simulink library "lib_controls"  (Simulink 7.9)
settings: Solver=ode45  SolverMode=SingleTasking  StartTime=0.0  StopTime=10.0  RelTol=1e-3
undefined symbols (not defined in the file or in its folder): amb_tmp, cs_charge_deplete_bool, cs_charge_pwr, cs_charge_trq, cs_clt_tmp, cs_decel_fc_off, cs_decel_regen_threshold, cs_dl_assist_trq_threshold, cs_dl_regen_trq_threshold, cs_electric_decel_spd, cs_electric_launch_spd, cs_electric_launch_spd_hi, cs_electric_launch_spd_lo, cs_eng_min_spd, cs_eng_on_soc, cs_fc_init_state, cs_fc_max_pwr_frac, cs_fc_min_pwr_frac, cs_fc_on, cs_fc_pwr_opt, cs_fc_spd_opt, cs_fuzzy_fuel_mode, cs_hi_soc, cs_hi_trq_frac, cs_lo_soc, cs_lo_trq_frac, cs_max_gc_spd, cs_max_pwr, cs_max_pwr_fall_rate, cs_max_pwr_rise_rate, cs_mc_assist_max_frac, cs_mc_assist_min_frac, cs_mc_assist_slope, cs_mc_regen_max_frac, cs_mc_regen_min_frac, cs_mc_regen_slope, cs_mean_eff, cs_mean_eff_bool, cs_min_gc_spd, cs_min_off_time, cs_min_pwr, cs_min_trq_frac, cs_mph_avg_time, cs_off_trq_frac, cs_plot_output, cs_pwr, cs_regen_avg_time, cs_scale_factor, cs_shutoff, cs_soc_range, cs_spd, cs_target_soc, cs_trq_to_soc_factor, cvt_locus_pwr, cvt_locus_spd, cyc_mph, enable_sim_stop_distance, enable_sim_stop_max_spd, enable_sim_stop_speed, enable_sim_stop_time ... (+110)
libraries: lib_controls x124, simulink3 x13, simulink x5, lib_etc x1
(part 1 of 17)
settings Model: Creator=mokeefe  LastModifiedBy=mokeefe
settings Model: ModifiedComment=|
  | mokeefe -- Fri Mar 23 16:02:54 2012 -- Version 1.480
  | Updated all instances of @1 variables in key-on block masks to use the variable name ("t" in all cases).
settings Model: ModifiedHistory=|
  | mokeefe -- Fri Mar 23 16:02:54 2012 -- Version 1.480
  | Updated all instances of @1 variables in key-on block masks to use the variable name ("t" in all cases).
  | 
  | mokeefe -- Fri Mar 23 15:55:42 2012 -- Version 1.479
  | Fixed mask issues -- key_on @1 to "t"
  | 
  | mokeefe -- Fri Mar 23 15:20:48 2012 -- Version 1.478
  | updated maks variable from @1 to variable name.
  | 
  | mokeefe -- Fri Mar 23 14:57:12 2012 -- Version 1.477
  | 
  | 
  | mokeefe -- Fri Mar 23 14:56:40 2012 -- Version 1.476
  | Updated <vc> conv cvt/engine control/key_on mask initialization from @1 to variable name.
  | 
  | mokeefe -- Fri Mar 23 14:35:59 2012 -- Version 1.475
  | Updated mask variable from @1 to variable name.
  | 
  | mokeefe -- Fri Mar 23 09:48:31 2012 -- Version 1.474
  | Fixed MaskInitiation string of block 'engine control/key_on' which used mask variables by reference (@1) vs by variable name.
  | 
  | ssprik -- Fri Oct 10 08:40:34 2003 -- Version 1.473
  | added goto tag for F_rear_brake_req
  | 
  | ssprik -- Thu Oct 09 15:11:40 2003 -- Version 1.472
  | added F_rear_brake_req   goto
  | 
  | tmarkel -- Fri Mar 07 09:53:07 2003 -- Version 1.471
  | 
  | added logic to allow user to keep the engine on during a drive cycle unless the key if off or the engine has been manually disabled
  | 
  | tmarkel -- Fri Mar 07 09:43:58 2003 -- Version 1.470
  | 
  | added an override bool to keep engine on at all times
  | 
  | 
  | tmarkel -- Mon Mar 03 14:14:43 2003 -- Version 1.469
  | 
  | updated traction control block in all vehicle control blocks to 2 axle version
  | 
  | tmarkel -- Mon Mar 03 14:07:59 2003 -- Version 1.468
  | 
  | added output from blocks for rear params from traction blocks in all vehicle control blocks
  | 
  | temp solution - added grounds as inputs to the brake controller for rear drivetrain output to eliminate warnings
  | 
  | 
  | 
  | 
  | tmarkel -- Mon Mar 03 12:40:46 2003 -- Version 1.467
  | 
  | 
  | tmarkel -- Mon Mar 03 12:37:51 2003 -- Version 1.466
  | removed extra traction control model from conv.
  | 
  | tmarkel -- Mon Mar 03 12:29:10 2003 -- Version 1.465
  | 
  | updated traction control config subsystem to be two axle model
  | 
  | tmarkel -- Mon Feb 24 16:12:37 2003 -- Version 1.464
  | updated j2452 model for 2 axles
  | 
  | abrooker -- Thu Feb 20 14:21:28 2003 -- Version 1.463
  | 
  | 
  | mokeefe -- Wed Feb 19 08:45:17 2003 -- Version 1.462
  | 
  | 
  | mokeefe -- Wed Feb 19 08:43:58 2003 -- Version 1.461
  | 
  | 
  | tmarkel -- Fri Feb 14 10:10:01 2003 -- Version 1.460
  | 
  | 
  | tmarkel -- Fri Feb 14 10:08:23 2003 -- Version 1.459
  | 
  | 
  | tmarkel -- Thu Feb 13 12:55:41 2003 -- Version 1.458
  | 
  | 
  | tmarkel -- Thu Feb 13 12:32:44 2003 -- Version 1.457
  | 
  | 
  | tmarkel -- Wed Feb 12 15:47:27 2003 -- Version 1.456
  | fixed one more broken link
  | 
  | tmarkel -- Wed Feb 12 15:29:50 2003 -- Version 1.455
  | updated conv controller to include front/rear traction model
  | 
  | 
  | tmarkel -- Wed Feb 12 15:07:56 2003 -- Version 1.454
  | fixed broken link to lib_controls_2axle
  | 
  | tmarkel -- Wed Feb 12 14:32:44 2003 -- Version 1.453
  | fixed bad link errors
  | 
  | tmarkel -- Wed Feb 12 09:39:27 2003 -- Version 1.452
  | 
  | Added the traction control blocks for a front/rear traction system to the subsystem box
  | 
  | 
  | bjeanner -- Thu Dec 26 09:42:29 2002 -- Version 1.451
  | add three new parameters: allowing calcultion of equivallent ESS function with mean efficiency; plus plotting results parameter
  | 
  | 
  | bjeanner -- Thu Dec 12 14:52:52 2002 -- Version 1.450
  | 
  | 
  | bjeanner -- Tue Dec 10 14:49:05 2002 -- Version 1.449
  | 
  | 
  | bjeanner -- Tue Dec 10 13:14:31 2002 -- Version 1.448
  | 
  | 
  | bjeanner -- Tue Dec 10 11:50:56 2002 -- Version 1.447
  | 
  | 
  | bjeanner -- Tue Dec 10 11:41:01 2002 -- Version 1.446
  | 
  | 
  | bjeanner -- Tue Dec 10 11:30:40 2002 -- Version 1.445
  | 
  | 
  | bjeanner -- Tue Dec 10 11:29:40 2002 -- Version 1.444
  | 
  | 
  | bjeanner -- Tue Dec 10 11:10:40 2002 -- Version 1.443
  | 
  | 
  | bjeanner -- Tue Dec 10 10:31:25 2002 -- Version 1.442
  | 
  | 
  | bjeanner -- Tue Dec 10 10:30:04 2002 -- Version 1.441
  | 
  | 
  | bjeanner -- Tue Dec 10 10:29:36 2002 -- Version 1.440
  | 
  | 
  | bjeanner -- Tue Dec 10 10:23:30 2002 -- Version 1.439
  | 
  | 
  | bjeanner -- Tue Dec 10 09:20:40 2002 -- Version 1.438
  | 
  | 
  | bjeanner -- Tue Dec 10 09:16:26 2002 -- Version 1.437
  | Add the template for the configurable subsystem for the BD_FUELCELL control strategy.
  | Add the fuel cell adaptive control strategy
  | 
  | 
  | mokeefe -- Tue Aug 13 07:36:17 2002 -- Version 1.436
  | Making the model look "pretty"
  | 
  | mokeefe -- Tue Aug 13 07:35:11 2002 -- Version 1.435
  | changed <vc> conv cvt/cvt control to use "acc_mech_pwr_est" instead of "acc_mech_trq_est" as had been used previously (the required datum is the power and not the torque!)
  | 
  | ssprik -- Tue Apr 30 11:21:35 2002 -- Version 1.434
  | added user contributed par bal engine on  block
  | 
  | mokeefe -- Tue Apr 23 09:06:10 2002 -- Version 1.433
  | changed Insight electric assist control strategy <cs> DIRECT SPLIT/Hard Acceleration to prevent a divide by zero warning. Also added logic to prevent a torque request above the maximum achievable motor torque.
  | 
  | mokeefe -- Tue Apr 23 09:03:51 2002 -- Version 1.432
  | changed Insight electric assist control strategy <cs> DIRECT SPLIT/Hard Acceleration to prevent a divide by zero warning. Also added logic to prevent a torque request above the maximum achievable motor torque.
  | 
  | mokeefe -- Tue Apr 23 08:50:58 2002 -- Version 1.431
  | 
  | 
  | ssprik -- Thu Apr 18 14:34:50 2002 -- Version 1.430
  | 
  | 
  | ssprik -- Thu Apr 18 14:32:52 2002 -- Version 1.429
  | 
  | 
  | ssprik -- Thu Apr 18 14:06:57 2002 -- Version 1.428
  | 
  | 
  | ssprik -- Thu Apr 18 13:56:10 2002 -- Version 1.427
  | 
  | 
  | ssprik -- Thu Apr 18 13:46:32 2002 -- Version 1.426
  | 
  | 
  | kkelly -- Thu Apr 18 10:17:40 2002 -- Version 1.425
  | 
  | 
  | mokeefe -- Thu Apr 18 08:23:32 2002 -- Version 1.424
  | saving the model:
  | o "without the model browser open"
  | o with only top-level screen visible
  | o with "fit to view" enabled
  | o with "status bar" off and "toolbar" off
  | o with "prompt to update model history with each save" on
  | 
  | kkelly -- Wed Mar 27 14:57:12 2002 -- Version 1.423
  | 
  | 
  | kkelly -- Wed Mar 27 14:57:12 2002 -- Version 1.423
  | 
  | 
  | kkelly -- Wed Mar 27 14:50:41 2002 -- Version 1.422
  | 
  | 
  | kkelly -- Wed Mar 27 14:50:24 2002 -- Version 1.421
  | 
  | 
  | kkelly -- Wed Mar 27 14:26:31 2002 -- Version 1.420
  | 
  | 
  | kkelly -- Wed Mar 27 14:26:16 2002 -- Version 1.419
  | 
  | 
  | kkelly -- Wed Mar 27 14:25:54 2002 -- Version 1.418
  | 
  | 
  | kkelly -- Wed Mar 27 14:20:49 2002 -- Version 1.417
  | 
  | 
  | kkelly -- Wed Mar 27 14:18:25 2002 -- Version 1.416
  | 
  | 
  | kkelly -- Wed Mar 27 14:17:14 2002 -- Version 1.415
  | 
  | 
  | kkelly -- Wed Mar 27 14:09:18 2002 -- Version 1.414
  | 
  | 
  | kkelly -- Wed Mar 27 14:07:10 2002 -- Version 1.413
  | 
  | 
  | kkelly -- Wed Mar 27 14:04:42 2002 -- Version 1.412
  | 
  | 
  | kkelly -- Wed Mar 27 12:39:55 2002 -- Version 1.411
  | 
  | 
  | kkelly -- Wed Mar 27 12:39:35 2002 -- Version 1.410
  | 
  | 
  | kkelly -- Wed Mar 27 12:31:18 2002 -- Version 1.409
  | 
  | 
  | kkelly -- Wed Mar 27 12:12:25 2002 -- Version 1.408
  | 
  | 
  | kkelly -- Wed Mar 27 12:03:57 2002 -- Version 1.407
  | 
  | 
  | kkelly -- Wed Mar 27 12:03:11 2002 -- Version 1.406
  | Added logic to increase torque request for very hard acceleration
  | 
  | kkelly -- Wed Mar 27 11:51:32 2002 -- Version 1.405
  | Added logic to allow EM in 1st gear when torque request is high
  | 
  | kkelly -- Wed Mar 27 11:48:18 2002 -- Version 1.404
  | Added logic to allow EM at low speed with high torque request
  | 
  | kkelly -- Wed Mar 27 11:36:20 2002 -- Version 1.403
  | Added zero-torque request logic
  | 
  | kkelly -- Wed Mar 27 11:09:35 2002 -- Version 1.402
  | 
  | 
  | kkelly -- Wed Mar 27 11:07:39 2002 -- Version 1.401
  | 
  | 
  | kkelly -- Wed Mar 27 10:43:33 2002 -- Version 1.400
  | 
  | 
  | mokeefe -- Fri Mar 08 08:11:28 2002 -- Version 1.399
  | took all separate auxiliary load calculations out of the <vc> libraries. These will now use the lib_accessory goto tags (acc_mech_trq_est, acc_mech_pwr_est, acc_elec_pwr_est)
  | 
  | mokeefe -- Mon Jul 02 10:08:55 2001 -- Version 1.184
  | 
  | 
  | mokeefe -- Mon Jul 02 10:08:07 2001 -- Version 1.183
  | 
  | 
  | mokeefe -- Mon Jul 02 10:06:51 2001 -- Version 1.182
  | 
  | 
  | mokeefe -- Mon Jul 02 10:05:17 2001 -- Version 1.181
  | 
  | 
  | mokeefe -- Mon Jul 02 10:04:17 2001 -- Version 1.180
  | 
  | 
  | mokeefe -- Fri Jun 29 13:59:18 2001 -- Version 1.179
  | 
  | all <vc> blocks updated for use with variable cargo mass functionality (cargo mass by distance)--also, all <vc> top-level blocks have been "cleaned up" to look neat and organized. A sub-model library has been made and is the preferred way to do future development.
  | 
  | mokeefe -- Fri Jun 29 13:56:37 2001 -- Version 1.178
  | 
  | <vc> prius
  | 
  | mokeefe -- Fri Jun 29 13:46:29 2001 -- Version 1.177
  | 
  | 
  | mokeefe -- Fri Jun 29 13:40:43 2001 -- Version 1.176
  | 
  | 
  | mokeefe -- Fri Jun 29 13:39:38 2001 -- Version 1.175
  | 
  | <vc> series ("" "")
  | 
  | 
  | mokeefe -- Fri Jun 29 13:34:00 2001 -- Version 1.174
  | 
  | <vc> par Adaptive ("" "")
  | 
  | mokeefe -- Fri Jun 29 13:23:41 2001 -- Version 1.173
  | 
  | insight (ibid.)
  | 
  | 
  | mokeefe -- Fri Jun 29 13:15:22 2001 -- Version 1.172
  | 
  | <vc> par balanced--> veh_mass to veh_mass+veh_cargo_mass
  | 
  | 
  | mokeefe -- Fri Jun 29 13:05:39 2001 -- Version 1.171
  | 
  | 
  | mokeefe -- Fri Jun 29 12:10:12 2001 -- Version 1.170
  | 
  | finished veh_mass mods for the <vc> par cvt...
  | 
  | 
  | mokeefe -- Fri Jun 29 12:09:18 2001 -- Version 1.169
  | 
  | 
  | mokeefe -- Fri Jun 29 11:56:20 2001 -- Version 1.168
  | 
  | 
  | mokeefe -- Fri Jun 29 11:44:30 2001 -- Version 1.167
  | 
  | 
  | mokeefe -- Fri Jun 29 11:33:07 2001 -- Version 1.166
  | 
  | 
  | mokeefe -- Fri Jun 29 11:21:54 2001 -- Version 1.165
  | 
  | 
  | mokeefe -- Fri Jun 29 11:15:04 2001 -- Version 1.164
  | 
  | 
  | mokeefe -- Fri Jun 29 11:13:02 2001 -- Version 1.163
  | 
  | 
  | mokeefe -- Fri Jun 29 11:06:47 2001 -- Version 1.162
  | 
  | 
  | mokeefe -- Fri Jun 29 11:04:27 2001 -- Version 1.161
  | 
  | 
  | mokeefe -- Fri Jun 29 10:40:33 2001 -- Version 1.160
  | 
  | 
  | mokeefe -- Fri Jun 29 10:35:18 2001 -- Version 1.159
  | 
  | 
  | mokeefe -- Fri Jun 29 10:29:06 2001 -- Version 1.158
  | 
  | 
  | mokeefe -- Fri Jun 29 10:26:50 2001 -- Version 1.157
  | 
  | 
  | mokeefe -- Fri Jun 29 10:18:10 2001 -- Version 1.156
  | 
  | made traction control, front and rear brake controller, and braking strategy into "sub-libraries" for vehicle control
  | 
  | mokeefe -- Fri Jun 29 10:17:11 2001 -- Version 1.155
  | 
  | 
  | mokeefe -- Fri Jun 29 10:15:46 2001 -- Version 1.154
  | 
  | 
  | mokeefe -- Fri Jun 29 10:09:48 2001 -- Version 1.153
  | 
  | 
  | mokeefe -- Fri Jun 29 09:58:42 2001 -- Version 1.152
  | 
  | 
  | mokeefe -- Fri Jun 29 09:57:37 2001 -- Version 1.151
  | 
  | creating sub-components for vehicle control model (traction control)
  | 
  | mokeefe -- Fri Jun 29 09:21:23 2001 -- Version 1.150
  | 
  | 
  | mokeefe -- Fri Jun 29 09:19:46 2001 -- Version 1.149
  | 
  | 
  | mokeefe -- Fri Jun 29 09:09:49 2001 -- Version 1.148
  | 
  | 
  | mokeefe -- Fri Jun 29 08:32:46 2001 -- Version 1.147
  | 
  | 
  | mokeefe -- Fri Jun 29 08:29:03 2001 -- Version 1.146
  | 
  | replacing veh_mass with veh_mass plus veh_cargo_mass in <vc> conv auto Saber Custom
  | 
  | 
  | mokeefe -- Thu Jun 28 17:08:40 2001 -- Version 1.145
  | 
  | 
  | mokeefe -- Thu Jun 28 17:07:02 2001 -- Version 1.144
  | 
  | 
  | mokeefe -- Thu Jun 28 17:06:28 2001 -- Version 1.143
  | 
  | changes to the CVT controls to subsitute veh_mass + veh_cargo_mass for veh_mass
  | 
  | 
  | mokeefe -- Thu Jun 28 16:55:42 2001 -- Version 1.142
  | 
  | 
  | mokeefe -- Thu Jun 28 16:32:01 2001 -- Version 1.141
  | 
  | changing veh_mass to veh_mass plus veh_cargo_mass
  | 
  | 
  | mokeefe -- Thu Jun 28 16:21:30 2001 -- Version 1.140
  | 
  | replacing veh_mass with veh_mass + (cargo mass vs time)
  | 
  | mokeefe -- Thu Jun 28 14:12:51 2001 -- Version 1.139
  | 
  | replaced all 'veh_mass' references with a veh_mass plus a FROM block (originating from drive cycle) that gives variable cargo mass by time

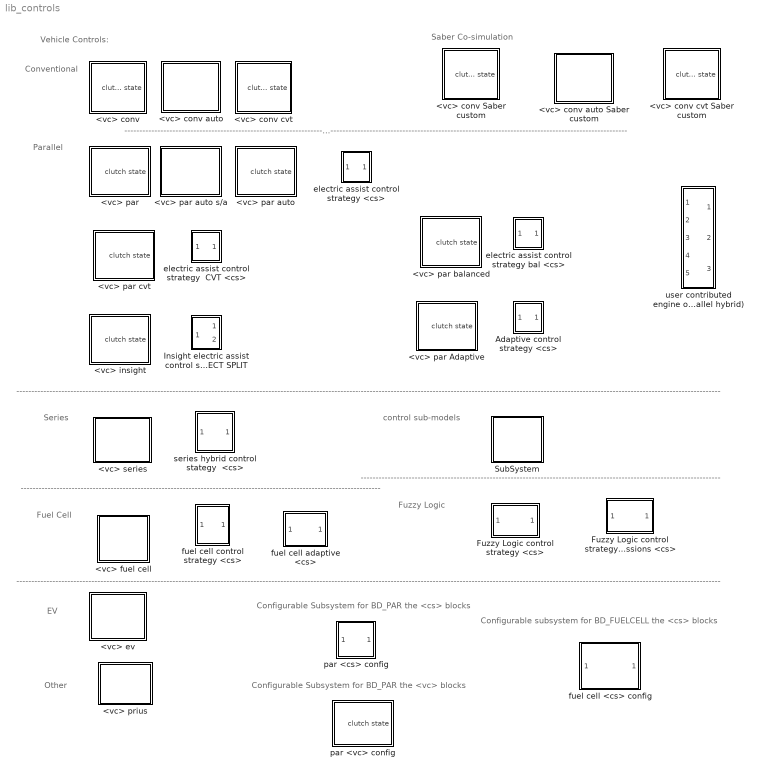
== system lib_controls ==
  note: Vehicle Controls:
  note: Conventional
  note: Series
  note: Parallel
  note: Fuel Cell
  note: EV
  note: Other
  note: ---------------------------------------------------------------------------------------------------------------------------------------------------------------------------------------------------------------------------------------------------------------------
  note: ------------------------------------------------------------------------------------------------------------------------
  note: ------------------------------------------------------------------------------------------------------------------------
  note: ------------------------------------------------------------------------------------------------------------------------
  note: ------------------------------------------------------------------------------------------------------------------------
  note: Saber Co-simulation
  note: control sub-models
  note: ------------------------------------------------------------------------------------------------------------------------
  note: Fuzzy Logic
  note: ------------------------------------------------------------------------------------------------------------------------
  note: Configurable Subsystem for BD_PAR the <cs> blocks
  note: Configurable Subsystem for BD_PAR the <vc> blocks
  note: Configurable subsystem for BD_FUELCELL the <cs> blocks
  <vc> conv : Subsystem
      mask Display: image(imread('bdi_vc.jpg'))
  <vc> conv Saber custom : Subsystem
      mask Display: image(imread('bdi_vc.jpg'))
  <vc> conv auto : Subsystem
      mask Display: image(imread('bdi_vc.jpg'))
  <vc> conv auto Saber custom : Subsystem
      mask Display: image(imread('bdi_vc.jpg'))
  <vc> conv cvt : Subsystem
      mask Display: image(imread('bdi_vc.jpg'))
  <vc> conv cvt Saber custom : Subsystem
      mask Display: image(imread('bdi_vc.jpg'))
  <vc> ev : Subsystem
      mask Display: image(imread('bdi_vc.jpg'))
  <vc> fuel cell : Subsystem
      mask Display: image(imread('bdi_vc.jpg'))
  <vc> insight : Subsystem
      mask Display: image(imread('bdi_vc.jpg'))
  <vc> par : Subsystem
      mask Display: image(imread('bdi_vc.jpg'))
  <vc> par Adaptive : Subsystem
      mask Display: image(imread('bdi_vc.jpg'))
  <vc> par auto : Subsystem
      mask Display: image(imread('bdi_vc.jpg'))
  <vc> par auto s/a : Subsystem
      mask Display: image(imread('bdi_vc.jpg'))
  <vc> par balanced : Subsystem
      mask Display: image(imread('bdi_vc.jpg'))
  <vc> par cvt : Subsystem
      mask Display: image(imread('bdi_vc.jpg'))
  <vc> prius : Subsystem
      mask Display: image(imread('bdi_vc.jpg'))
  <vc> series : Subsystem
      mask Display: image(imread('bdi_vc.jpg'))
  Adaptive control strategy <cs> : Subsystem
      mask Display: image(imread('bdi_cs.jpg'))
  Fuzzy Logic control strategy <cs> : Subsystem
      mask Description:
      | This Block contains the Fuzzy Logic Control Strategy to control a parallel hybird configuration. 2 modes of operation are available.
      | 
      | A FUEL USE mode limits the instantaneous fuel use of the IC engine.
      | An EFFICIENCY mode tries to operate the IC engine near regions of peak efficiency.
      | 
      | To look at the CONTENTS of this block, right-click and choose "Look under Mask".
      mask Display: image(imread('bdi_fuzzy.jpg'))
  Fuzzy Logic control strategy with Emissions <cs> : Subsystem
      mask Display: image(imread('bdi_fuzzy.jpg'))
  Insight electric assist control strategy <cs> DIRECT SPLIT : Subsystem  AncestorBlock=|
      | lib_controls/Insight electric assist
      | control strategy
      | <cs> DIRECT SPLIT
      mask Display: image(imread('bdi_cs.jpg'))
  SubSystem : Subsystem
  electric assist control strategy <cs> : Subsystem
      mask Display: image(imread('bdi_cs.jpg'))
  electric assist control strategy bal <cs> : Subsystem
      mask Display: image(imread('bdi_cs.jpg'))
  electric assist control strategy  CVT <cs> : Subsystem
      mask Display: image(imread('bdi_cs.jpg'))
  fuel cell adaptive <cs> : Subsystem
      mask Display: image(imread('bdi_cs.jpg'))
  fuel cell control strategy <cs> : Subsystem
      mask Display: image(imread('bdi_cs.jpg'))
  fuel cell <cs> config : Subsystem  BlockChoice=fuel cell adaptive <cs>
      settings: TemplateBlock=self  MemberBlocks=fuel cell adaptive <cs>,fuel cell control strategy <cs>
  par <cs> config : Subsystem  BlockChoice=electric assist control strategy <cs>
      settings: TemplateBlock=self  MemberBlocks=Adaptive control strategy <cs>,Fuzzy Logic control strategy <cs>,Fuzzy Logic control strategy with Emissions <cs>,electric assist control strategy <cs>,electric assist control strategy bal <cs>
  par <vc> config : Subsystem  BlockChoice=<vc> par
      settings: TemplateBlock=self  MemberBlocks=<vc> par,<vc> par Adaptive,<vc> par balanced
  series hybrid control stategy  <cs> : Subsystem
      mask Display: image(imread('bdi_cs.jpg'))
  user contributed engine on (balanced parallel hybrid) : Subsystem  AncestorBlock=|
      | lib_controls/<vc> ISG bal shift
      | by time CD3xx/engine on
      | (balanced parallel hybrid)

== system lib_controls/<vc> conv ==
  note: required force (N)
  Relational Operator : RelationalOperator  Operator=~=  InputSameDT=on
  Sum : Sum  Inputs=-+  SaturateOnIntegerOverflow=on  InputSameDT=on  OutDataTypeStr=Inherit: Same as first input
  braking strategy : lib_controls/SubSystem/braking strategy
  clutch control : Subsystem
  config traction control : Subsystem  BlockChoice=traction control 2 axle
      settings: AttributesFormatString=%<BlockChoice>  TemplateBlock=lib_controls/SubSystem/config traction control  MemberBlocks=traction control 2 axle,traction control J2452 2 axle
  engine control : Subsystem
  front and rear brake controller (achievable) : lib_controls/SubSystem/front and rear brake controller (achievable)
  gearbox  control : Subsystem
  sim stop subsystem : lib_controls/SubSystem/sim stop subsystem
  clutch state : Outport
  tag scope: F_front_brake=global, F_front_brake_req=global, F_rear_brake=global, F_rear_brake_req=global, F_req_limited=global, clutch_state=global, engine_on=global, front_traction_ratio=global, gear_number=global, gear_ratio=global, key_on=global, shifting=global, slip_limited=global, spd_command=global, v_req_limited=global, wt_front_axle=global, wt_rear_axle=global
  wires:
  engine control/3(key on) -> [key_on]
  engine control/1(engine on) -> [engine_on]
  engine control/2(spd command  (rad/s)) -> [spd_command]
  [fc_spd_out_r] -> engine control/3(fc_spd_out_r)
  [shifting] -> engine control/2(shifting)
  [clutch_state] -> engine control/1(clutch state)
  [v_ave_req] -> engine control/4(v_ave_req)
  clutch control/1(clutch state) -> [clutch_state], clutch state/1
  [w_cl_out] -> clutch control/3(gb_spd_in_r)
  [T_cl_out] -> clutch control/2(gb_trq_in_r)
  [shifting] -> clutch control/1(shifting)
  gearbox  control/1("gear ratio, out") -> [gear_ratio]
  [T_gb_out] -> gearbox  control/1(gb_trq_out_r)
  [w_gb_out] -> gearbox  control/2(gb_spd_out_r)
  [eta_gb] -> gearbox  control/3(prev. Pout/Pin)
  [slip_limited] -> gearbox  control/4(tires are at traction limit)
  gearbox  control/2("shifting, out") -> [shifting]
  front and rear brake controller (achievable)/1 -> [F_front_brake]
  [F_drivetrain_ach] -> front and rear brake controller (achievable)/2
  [w_wheel_ach] -> front and rear brake controller (achievable)/3
  [F_max_front_brake] -> front and rear brake controller (achievable)/4
  [F_max_rear_brake] -> front and rear brake controller (achievable)/5
  front and rear brake controller (achievable)/2 -> [F_rear_brake]
  [F_req] -> front and rear brake controller (achievable)/1
  braking strategy/2 -> Sum/1, [F_rear_brake_req]
  config traction control/1(req'd force (N)) -> braking strategy/2, Sum/2, Relational Operator/1
  braking strategy/1 -> [F_front_brake_req]
  [v_prev] -> config traction control/2(vehicle speed at beginning of time  step (m/s))
  config traction control/3(weight on front axle (N)) -> [wt_front_axle]
  [F_req] -> config traction control/3(total tractive force req'd (N))
  Sum/1 -> [F_req_limited]
  Relational Operator/1 -> [slip_limited]
  [F_req] -> Relational Operator/2
  [v_ave_req] -> config traction control/1(time-average vehicle speed  req'd (m/s))
  [v_ave_req] -> braking strategy/1
  gearbox  control/3("gear number, out") -> [gear_number]
  config traction control/2(req'd speed (m/s)) -> [v_req_limited]
  config traction control/4(weight on rear axle (N)) -> [wt_rear_axle]
  config traction control/5(front/total  traction ratio) -> [front_traction_ratio]
  [F_rear_drivetrain_ach] -> front and rear brake controller (achievable)/6

== system lib_controls/<vc> conv Saber custom ==
  Ground : Ground
  Relational Operator : RelationalOperator  Operator=~=  InputSameDT=on
  Sum : Sum  Inputs=-+  SaturateOnIntegerOverflow=on  InputSameDT=on  OutDataTypeStr=Inherit: Same as first input
  braking strategy : lib_controls/SubSystem/braking strategy
  clutch control : Subsystem
  config traction control : Subsystem  BlockChoice=traction control 2 axle
      settings: AttributesFormatString=%<BlockChoice>  TemplateBlock=lib_controls/SubSystem/config traction control  MemberBlocks=traction control 2 axle,traction control J2452 2 axle
  engine control : Subsystem
  front and rear brake controller (achievable) : lib_controls/SubSystem/front and rear brake controller (achievable)
  gearbox  control : Subsystem
  sim stop subsystem : lib_controls/SubSystem/sim stop subsystem
  clutch state : Outport
  tag scope: F_front_brake=global, F_front_brake_req=global, F_rear_brake=global, F_rear_brake_req=global, F_req_limited=global, clutch_state=global, engine_on=global, front_traction_ratio=global, gear_number=global, gear_ratio=global, key_on=global, shifting=global, slip_limited=global, spd_command=global, v_req_limited=global, wt_front_axle=global, wt_rear_axle=global
  wires:
  front and rear brake controller (achievable)/2 -> [F_rear_brake]
  [F_max_rear_brake] -> front and rear brake controller (achievable)/5
  [F_max_front_brake] -> front and rear brake controller (achievable)/4
  [w_wheel_ach] -> front and rear brake controller (achievable)/3
  [F_drivetrain_ach] -> front and rear brake controller (achievable)/2
  front and rear brake controller (achievable)/1 -> [F_front_brake]
  [F_req] -> front and rear brake controller (achievable)/1
  [eta_gb] -> gearbox  control/3(prev. Pout/Pin)
  [w_gb_out] -> gearbox  control/2(gb_spd_out_r)
  [T_gb_out] -> gearbox  control/1(gb_trq_out_r)
  [slip_limited] -> gearbox  control/4(tires are at traction limit)
  config traction control/3(weight on front axle (N)) -> [wt_front_axle]
  config traction control/2(req'd speed (m/s)) -> [v_req_limited]
  [v_prev] -> config traction control/2(vehicle speed at beginning of time  step (m/s))
  braking strategy/1 -> [F_front_brake_req]
  config traction control/1(req'd force (N)) -> braking strategy/2, Sum/2, Relational Operator/1
  braking strategy/2 -> Sum/1, [F_rear_brake_req]
  [F_req] -> config traction control/3(total tractive force req'd (N))
  Sum/1 -> [F_req_limited]
  Relational Operator/1 -> [slip_limited]
  [F_req] -> Relational Operator/2
  [v_ave_req] -> config traction control/1(time-average vehicle speed  req'd (m/s))
  [v_ave_req] -> braking strategy/1
  [T_cl_out] -> clutch control/2(gb_trq_in_r)
  [w_cl_out] -> clutch control/3(gb_spd_in_r)
  clutch control/1(clutch state) -> [clutch_state], clutch state/1
  [shifting] -> clutch control/1(shifting)
  [fc_spd_out_r] -> engine control/3(fc_spd_out_r)
  engine control/2(spd command  (rad/s)) -> [spd_command]
  engine control/1(engine on) -> [engine_on]
  engine control/3(key on) -> [key_on]
  [v_ave_req] -> engine control/4(v_ave_req)
  [shifting] -> engine control/2(shifting)
  [clutch_state] -> engine control/1(clutch state)
  gearbox  control/3("gear number, out") -> [gear_number]
  gearbox  control/2("shifting, out") -> [shifting]
  gearbox  control/1("gear ratio, out") -> [gear_ratio]
  config traction control/4(weight on rear axle (N)) -> [wt_rear_axle]
  config traction control/5(front/total  traction ratio) -> [front_traction_ratio]
  Ground/1 -> front and rear brake controller (achievable)/6

== system lib_controls/<vc> conv auto ==
  note: required
      | force (N)
  Constant : Constant  Value=3
  Ground : Ground
  Relational Operator : RelationalOperator  Operator=~=  InputSameDT=on
  Sum : Sum  Inputs=-+  SaturateOnIntegerOverflow=on  InputSameDT=on  OutDataTypeStr=Inherit: Same as first input
  braking strategy : lib_controls/SubSystem/braking strategy
  config traction control : Subsystem  BlockChoice=traction control 2 axle
      settings: AttributesFormatString=%<BlockChoice>  TemplateBlock=lib_controls/SubSystem/config traction control  MemberBlocks=traction control 2 axle,traction control J2452 2 axle
  engine control : Subsystem
  front and rear brake controller (achievable) : lib_controls/SubSystem/front and rear brake controller (achievable)
  gearbox control for use w/ AT : Subsystem
  sim stop subsystem : lib_controls/SubSystem/sim stop subsystem
  tag scope: F_front_brake=global, F_front_brake_req=global, F_rear_brake=global, F_rear_brake_req=global, F_req_limited=global, clutch_state=global, engine_on=global, front_traction_ratio=global, gear_number=global, gear_ratio=global, key_on=global, locked_up=global, shifting=global, slip_limited=global, spd_command=global, v_req_limited=global, wt_front_axle=global, wt_rear_axle=global
  wires:
  front and rear brake controller (achievable)/2 -> [F_rear_brake]
  [F_max_rear_brake] -> front and rear brake controller (achievable)/5
  [F_max_front_brake] -> front and rear brake controller (achievable)/4
  [w_wheel_ach] -> front and rear brake controller (achievable)/3
  [F_drivetrain_ach] -> front and rear brake controller (achievable)/2
  front and rear brake controller (achievable)/1 -> [F_front_brake]
  [F_req] -> front and rear brake controller (achievable)/1
  engine control/2(spd command  (rad/s)) -> [spd_command]
  [fc_spd_out_r] -> engine control/3(fc_spd_out_r)
  engine control/1(engine on) -> [engine_on]
  engine control/3(key on) -> [key_on]
  [v_ave_req] -> engine control/4(v_ave_req)
  [clutch_state] -> engine control/2(clutch state)
  [shifting] -> engine control/1(shifting)
  Constant/1 -> [clutch_state]
  gearbox control for use w/ AT/4(locked up) -> [locked_up]
  gearbox control for use w/ AT/2("gear ratio, out") -> [gear_ratio]
  gearbox control for use w/ AT/1("gear number, out") -> [gear_number]
  [eta_gb] -> gearbox control for use w/ AT/1(eta_gb)
  [slip_limited] -> gearbox control for use w/ AT/4(tires are at traction limit)
  [T_gb_out] -> gearbox control for use w/ AT/2(gb_trq_out_r)
  [w_gb_out] -> gearbox control for use w/ AT/3(gb_spd_out_r)
  gearbox control for use w/ AT/3("shifting, out") -> [shifting]
  Sum/1 -> [F_req_limited]
  Relational Operator/1 -> [slip_limited]
  config traction control/3(weight on front axle (N)) -> [wt_front_axle]
  config traction control/2(req'd speed (m/s)) -> [v_req_limited]
  [v_prev] -> config traction control/2(vehicle speed at beginning of time  step (m/s))
  config traction control/1(req'd force (N)) -> braking strategy/2, Sum/2, Relational Operator/1
  [F_req] -> config traction control/3(total tractive force req'd (N))
  [v_ave_req] -> config traction control/1(time-average vehicle speed  req'd (m/s))
  braking strategy/1 -> [F_front_brake_req]
  braking strategy/2 -> Sum/1, [F_rear_brake_req]
  [v_ave_req] -> braking strategy/1
  [F_req] -> Relational Operator/2
  Ground/1 -> front and rear brake controller (achievable)/6
  config traction control/5(front/total  traction ratio) -> [front_traction_ratio]
  config traction control/4(weight on rear axle (N)) -> [wt_rear_axle]

== system lib_controls/<vc> conv auto Saber custom ==
  note: required
      | force (N)
  Constant : Constant  Value=3
  Ground : Ground
  Relational Operator : RelationalOperator  Operator=~=  InputSameDT=on
  Sum : Sum  Inputs=-+  SaturateOnIntegerOverflow=on  InputSameDT=on  OutDataTypeStr=Inherit: Same as first input
  braking strategy : lib_controls/SubSystem/braking strategy
  config traction control : Subsystem  BlockChoice=traction control 2 axle
      settings: AttributesFormatString=%<BlockChoice>  TemplateBlock=lib_controls/SubSystem/config traction control  MemberBlocks=traction control 2 axle,traction control J2452 2 axle
  engine control : Subsystem
  front and rear brake controller (achievable) : lib_controls/SubSystem/front and rear brake controller (achievable)
  gearbox control for use w/ AT : Subsystem
  sim stop subsystem : lib_controls/SubSystem/sim stop subsystem
  tag scope: F_front_brake=global, F_front_brake_req=global, F_rear_brake=global, F_rear_brake_req=global, F_req_limited=global, clutch_state=global, engine_on=global, front_traction_ratio=global, gear_number=global, gear_ratio=global, key_on=global, locked_up=global, shifting=global, slip_limited=global, spd_command=global, v_req_limited=global, wt_front_axle=global, wt_rear_axle=global
  wires:
  front and rear brake controller (achievable)/1 -> [F_front_brake]
  [F_drivetrain_ach] -> front and rear brake controller (achievable)/2
  [w_wheel_ach] -> front and rear brake controller (achievable)/3
  [F_max_front_brake] -> front and rear brake controller (achievable)/4
  [F_max_rear_brake] -> front and rear brake controller (achievable)/5
  front and rear brake controller (achievable)/2 -> [F_rear_brake]
  [F_req] -> front and rear brake controller (achievable)/1
  [w_gb_out] -> gearbox control for use w/ AT/3(gb_spd_out_r)
  [T_gb_out] -> gearbox control for use w/ AT/2(gb_trq_out_r)
  [slip_limited] -> gearbox control for use w/ AT/4(tires are at traction limit)
  [eta_gb] -> gearbox control for use w/ AT/1(eta_gb)
  gearbox control for use w/ AT/4(locked up) -> [locked_up]
  engine control/3(key on) -> [key_on]
  engine control/1(engine on) -> [engine_on]
  [fc_spd_out_r] -> engine control/3(fc_spd_out_r)
  engine control/2(spd command  (rad/s)) -> [spd_command]
  [clutch_state] -> engine control/2(clutch state)
  [shifting] -> engine control/1(shifting)
  Constant/1 -> [clutch_state]
  [v_ave_req] -> engine control/4(v_ave_req)
  Relational Operator/1 -> [slip_limited]
  braking strategy/2 -> Sum/1, [F_rear_brake_req]
  config traction control/1(req'd force (N)) -> braking strategy/2, Sum/2, Relational Operator/1
  braking strategy/1 -> [F_front_brake_req]
  [v_prev] -> config traction control/2(vehicle speed at beginning of time  step (m/s))
  config traction control/2(req'd speed (m/s)) -> [v_req_limited]
  config traction control/3(weight on front axle (N)) -> [wt_front_axle]
  Sum/1 -> [F_req_limited]
  [F_req] -> config traction control/3(total tractive force req'd (N))
  [F_req] -> Relational Operator/2
  [v_ave_req] -> config traction control/1(time-average vehicle speed  req'd (m/s))
  [v_ave_req] -> braking strategy/1
  gearbox control for use w/ AT/1("gear number, out") -> [gear_number]
  gearbox control for use w/ AT/2("gear ratio, out") -> [gear_ratio]
  gearbox control for use w/ AT/3("shifting, out") -> [shifting]
  config traction control/4(weight on rear axle (N)) -> [wt_rear_axle]
  config traction control/5(front/total  traction ratio) -> [front_traction_ratio]
  Ground/1 -> front and rear brake controller (achievable)/6

== system lib_controls/<vc> conv cvt ==
  note: required
      | force (N)
  note: shifting is 0 (see above)
  note: note: shifting is "0", see above clutch cntrl
  Constant : Constant  Value=0
  Ground : Ground
  Relational Operator : RelationalOperator  Operator=~=  InputSameDT=on
  Sum : Sum  Inputs=-+  SaturateOnIntegerOverflow=on  InputSameDT=on  OutDataTypeStr=Inherit: Same as first input
  braking strategy : lib_controls/SubSystem/braking strategy
  clutch control : Subsystem
  config traction control : Subsystem  BlockChoice=traction control 2 axle
      settings: AttributesFormatString=%<BlockChoice>  TemplateBlock=lib_controls/SubSystem/config traction control  MemberBlocks=traction control 2 axle,traction control J2452 2 axle
  cvt control : Subsystem
  engine control : Subsystem
  front and rear brake controller (achievable) : lib_controls/SubSystem/front and rear brake controller (achievable)
  sim stop subsystem : lib_controls/SubSystem/sim stop subsystem
  clutch state : Outport
  tag scope: F_front_brake=global, F_front_brake_req=global, F_rear_brake=global, F_rear_brake_req=global, F_req_limited=global, clutch_state=global, engine_on=global, front_traction_ratio=global, gear_ratio=global, key_on=global, shifting=global, slip_limited=global, spd_command=global, v_req_limited=global, wt_front_axle=global, wt_rear_axle=global
  wires:
  config traction control/3(weight on front axle (N)) -> [wt_front_axle]
  config traction control/2(req'd speed (m/s)) -> [v_req_limited]
  [v_prev] -> config traction control/2(vehicle speed at beginning of time  step (m/s))
  config traction control/1(req'd force (N)) -> braking strategy/2, Sum/2, Relational Operator/1
  Sum/1 -> [F_req_limited]
  Relational Operator/1 -> [slip_limited]
  braking strategy/1 -> [F_front_brake_req]
  braking strategy/2 -> Sum/1, [F_rear_brake_req]
  [F_req] -> config traction control/3(total tractive force req'd (N))
  [F_req] -> Relational Operator/2
  [v_ave_req] -> config traction control/1(time-average vehicle speed  req'd (m/s))
  [v_ave_req] -> braking strategy/1
  front and rear brake controller (achievable)/2 -> [F_rear_brake]
  [F_max_rear_brake] -> front and rear brake controller (achievable)/5
  [F_max_front_brake] -> front and rear brake controller (achievable)/4
  [w_wheel_ach] -> front and rear brake controller (achievable)/3
  [F_drivetrain_ach] -> front and rear brake controller (achievable)/2
  front and rear brake controller (achievable)/1 -> [F_front_brake]
  [F_req] -> front and rear brake controller (achievable)/1
  cvt control/1("pulley ratio ") -> [gear_ratio]
  [eta_gb] -> cvt control/3(prev. Pout/Pin)
  [w_gb_out] -> cvt control/2(cvt_spd_out_r)
  [T_gb_out] -> cvt control/1(cvt_trq_out_r)
  [slip_limited] -> cvt control/4(tires are at traction limit)
  [T_cl_out] -> clutch control/2(gb_trq_in_r)
  [w_cl_out] -> clutch control/3(gb_spd_in_r)
  clutch control/1(clutch state) -> [clutch_state], clutch state/1
  engine control/1(engine on) -> [engine_on]
  engine control/2(spd command  (rad/s)) -> [spd_command]
  [fc_spd_out_r] -> engine control/3(fc_spd_out_r)
  engine control/3(key on) -> [key_on]
  [shifting] -> engine control/2(shifting)
  [clutch_state] -> engine control/1(clutch state)
  [shifting] -> clutch control/1(shifting)
  Constant/1 -> [shifting]
  [v_ave_req] -> engine control/4(v_ave_req)
  config traction control/4(weight on rear axle (N)) -> [wt_rear_axle]
  config traction control/5(front/total  traction ratio) -> [front_traction_ratio]
  Ground/1 -> front and rear brake controller (achievable)/6

== system lib_controls/<vc> conv cvt Saber custom ==
  note: required
      | force (N)
  Constant : Constant  Value=0
  Ground : Ground
  Relational Operator : RelationalOperator  Operator=~=  InputSameDT=on
  Sum : Sum  Inputs=-+  SaturateOnIntegerOverflow=on  InputSameDT=on  OutDataTypeStr=Inherit: Same as first input
  braking strategy : lib_controls/SubSystem/braking strategy
  clutch control : Subsystem
  config traction control : Subsystem  BlockChoice=traction control 2 axle
      settings: AttributesFormatString=%<BlockChoice>  TemplateBlock=lib_controls/SubSystem/config traction control  MemberBlocks=traction control 2 axle,traction control J2452 2 axle
  cvt control : Subsystem
  engine control : Subsystem
  front and rear brake controller (achievable) : lib_controls/SubSystem/front and rear brake controller (achievable)
  sim stop subsystem : lib_controls/SubSystem/sim stop subsystem
  clutch state : Outport
  tag scope: F_front_brake=global, F_front_brake_req=global, F_rear_brake=global, F_rear_brake_req=global, F_req_limited=global, clutch_state=global, engine_on=global, front_traction_ratio=global, gear_ratio=global, key_on=global, shifting=global, slip_limited=global, spd_command=global, v_req_limited=global, wt_front_axle=global, wt_rear_axle=global
  wires:
  Relational Operator/1 -> [slip_limited]
  braking strategy/2 -> Sum/1, [F_rear_brake_req]
  config traction control/1(req'd force (N)) -> braking strategy/2, Sum/2, Relational Operator/1
  braking strategy/1 -> [F_front_brake_req]
  [v_prev] -> config traction control/2(vehicle speed at beginning of time  step (m/s))
  config traction control/2(req'd speed (m/s)) -> [v_req_limited]
  config traction control/3(weight on front axle (N)) -> [wt_front_axle]
  engine control/3(key on) -> [key_on]
  [fc_spd_out_r] -> engine control/3(fc_spd_out_r)
  engine control/2(spd command  (rad/s)) -> [spd_command]
  engine control/1(engine on) -> [engine_on]
  clutch control/1(clutch state) -> [clutch_state], clutch state/1
  [w_cl_out] -> clutch control/3(gb_spd_in_r)
  [T_cl_out] -> clutch control/2(gb_trq_in_r)
  [v_ave_req] -> engine control/4(v_ave_req)
  [shifting] -> engine control/2(shifting)
  [clutch_state] -> engine control/1(clutch state)
  [shifting] -> clutch control/1(shifting)
  Constant/1 -> [shifting]
  [slip_limited] -> cvt control/4(tires are at traction limit)
  [T_gb_out] -> cvt control/1(cvt_trq_out_r)
  [w_gb_out] -> cvt control/2(cvt_spd_out_r)
  [eta_gb] -> cvt control/3(prev. Pout/Pin)
  cvt control/1("pulley ratio ") -> [gear_ratio]
  Sum/1 -> [F_req_limited]
  [F_req] -> config traction control/3(total tractive force req'd (N))
  [F_req] -> Relational Operator/2
  [v_ave_req] -> config traction control/1(time-average vehicle speed  req'd (m/s))
  [v_ave_req] -> braking strategy/1
  front and rear brake controller (achievable)/1 -> [F_front_brake]
  [F_drivetrain_ach] -> front and rear brake controller (achievable)/2
  [w_wheel_ach] -> front and rear brake controller (achievable)/3
  [F_max_front_brake] -> front and rear brake controller (achievable)/4
  [F_max_rear_brake] -> front and rear brake controller (achievable)/5
  front and rear brake controller (achievable)/2 -> [F_rear_brake]
  [F_req] -> front and rear brake controller (achievable)/1
  config traction control/4(weight on rear axle (N)) -> [wt_rear_axle]
  config traction control/5(front/total  traction ratio) -> [front_traction_ratio]
  Ground/1 -> front and rear brake controller (achievable)/6

== system lib_controls/<vc> ev ==
  note: force
      | required (N)
  Ground : Ground
  Relational Operator : RelationalOperator  Operator=~=  InputSameDT=on
  Sum : Sum  Inputs=-+  SaturateOnIntegerOverflow=on  InputSameDT=on  OutDataTypeStr=Inherit: Same as first input
  braking strategy : lib_controls/SubSystem/braking strategy
  config traction control : Subsystem  BlockChoice=traction control 2 axle
      settings: AttributesFormatString=%<BlockChoice>  TemplateBlock=lib_controls/SubSystem/config traction control  MemberBlocks=traction control 2 axle,traction control J2452 2 axle
  engaged : Constant  Value=3
  front and rear brake controller (achievable) : lib_controls/SubSystem/front and rear brake controller (achievable)
  gearbox control for series  HV and EV : Subsystem
  key_on : Subsystem  mask(Repeating table){t=vc_key_on(:,1), y=vc_key_on(:,2)}
      mask prompts: t "Time values:"; y "Output values:"
      mask help:
      | Repeating table.
      | Enter values of time and output for first cycle.
      mask init:
      | period = max(t);
      mask Help: Repeats cycle given in table. Time values should be monotonically increasing.
  motor controller logic : Subsystem
  sim stop subsystem : lib_controls/SubSystem/sim stop subsystem
  tag scope: F_front_brake=global, F_front_brake_req=global, F_rear_brake=global, F_rear_brake_req=global, F_req_limited=global, P_mc_in_r=global, clutch_state=global, front_traction_ratio=global, gear_number=global, gear_ratio=global, key_on=global, shifting=global, slip_limited=global, v_req_limited=global, wt_front_axle=global, wt_rear_axle=global
  wires:
  config traction control/3(weight on front axle (N)) -> [wt_front_axle]
  config traction control/2(req'd speed (m/s)) -> [v_req_limited]
  [v_prev] -> config traction control/2(vehicle speed at beginning of time  step (m/s))
  braking strategy/1 -> [F_front_brake_req]
  config traction control/1(req'd force (N)) -> braking strategy/2, Sum/2, Relational Operator/1
  braking strategy/2 -> Sum/1, [F_rear_brake_req]
  [w_mc_out_r] -> motor controller logic/4(req'd output spd (rad/s))
  [P_mc_in_1lim] -> motor controller logic/3(req'd input power (W))
  [bus_voltage] -> motor controller logic/2(bus voltage)
  motor controller logic/1(req'd input power (W)1) -> [P_mc_in_r]
  [shifting] -> motor controller logic/1(shifting)
  key_on/1(out_1) -> [key_on]
  [T_gb_out] -> gearbox control for series  HV and EV/1(gb_trq_out_r)
  [w_gb_out] -> gearbox control for series  HV and EV/2(gb_spd_out_r)
  [eta_gb] -> gearbox control for series  HV and EV/3(prev. Pout/Pin)
  [slip_limited] -> gearbox control for series  HV and EV/4(tires are at traction limit)
  engaged/1 -> [clutch_state]
  Sum/1 -> [F_req_limited]
  Relational Operator/1 -> [slip_limited]
  [F_req] -> Relational Operator/2
  [F_req] -> config traction control/3(total tractive force req'd (N))
  front and rear brake controller (achievable)/2 -> [F_rear_brake]
  [F_max_rear_brake] -> front and rear brake controller (achievable)/5
  [F_max_front_brake] -> front and rear brake controller (achievable)/4
  [w_wheel_ach] -> front and rear brake controller (achievable)/3
  [F_drivetrain_ach] -> front and rear brake controller (achievable)/2
  front and rear brake controller (achievable)/1 -> [F_front_brake]
  [F_req] -> front and rear brake controller (achievable)/1
  [v_ave_req] -> config traction control/1(time-average vehicle speed  req'd (m/s))
  [v_ave_req] -> braking strategy/1
  gearbox control for series  HV and EV/3("shifting, out") -> [shifting]
  gearbox control for series  HV and EV/2("gear ratio, out") -> [gear_ratio]
  gearbox control for series  HV and EV/1("gear number, out") -> [gear_number]
  config traction control/4(weight on rear axle (N)) -> [wt_rear_axle]
  config traction control/5(front/total  traction ratio) -> [front_traction_ratio]
  Ground/1 -> front and rear brake controller (achievable)/6

== system lib_controls/<vc> fuel cell ==
  Ground : Ground
  Relational Operator : RelationalOperator  Operator=~=  InputSameDT=on
  Sum : Sum  Inputs=-+  SaturateOnIntegerOverflow=on  InputSameDT=on  OutDataTypeStr=Inherit: Same as first input
  braking strategy : lib_controls/SubSystem/braking strategy
  config traction control : Subsystem  BlockChoice=traction control 2 axle
      settings: AttributesFormatString=%<BlockChoice>  TemplateBlock=lib_controls/SubSystem/config traction control  MemberBlocks=traction control 2 axle,traction control J2452 2 axle
  front and rear brake controller (achievable) : lib_controls/SubSystem/front and rear brake controller (achievable)
  gearbox control for series  HV and EV : Subsystem
  key_on : Subsystem  mask(Repeating table){t=vc_key_on(:,1), y=vc_key_on(:,2)}
      mask prompts: t "Time values:"; y "Output values:"
      mask help:
      | Repeating table.
      | Enter values of time and output for first cycle.
      mask init:
      | period = max(t);
      mask Help: Repeats cycle given in table. Time values should be monotonically increasing.
  motor controller logic : Subsystem
  series 'clutch' control : Subsystem
  sim stop subsystem : lib_controls/SubSystem/sim stop subsystem
  tag scope: F_front_brake=global, F_front_brake_req=global, F_rear_brake=global, F_rear_brake_req=global, F_req_limited=global, P_mc_in_r=global, clutch_state=global, front_traction_ratio=global, gear_number=global, gear_ratio=global, key_on=global, shifting=global, slip_limited=global, v_req_limited=global, wt_front_axle=global, wt_rear_axle=global
  wires:
  [w_mc_out_r] -> motor controller logic/3(req'd output spd (rad/s))
  [P_mc_in_1lim] -> motor controller logic/2(req'd input power (W))
  [bus_voltage] -> motor controller logic/1(bus voltage)
  motor controller logic/1(req'd input power (W)1) -> [P_mc_in_r]
  [shifting] -> motor controller logic/4(shifting)
  [slip_limited] -> gearbox control for series  HV and EV/4(tires are at traction limit)
  [T_gb_out] -> gearbox control for series  HV and EV/1(gb_trq_out_r)
  [w_gb_out] -> gearbox control for series  HV and EV/2(gb_spd_out_r)
  [eta_gb] -> gearbox control for series  HV and EV/3(prev. Pout/Pin)
  [engine_on] -> series 'clutch' control/1(engine on)
  series 'clutch' control/1(clutch state) -> [clutch_state]
  key_on/1(out_1) -> [key_on]
  config traction control/3(weight on front axle (N)) -> [wt_front_axle]
  config traction control/2(req'd speed (m/s)) -> [v_req_limited]
  [v_prev] -> config traction control/2(vehicle speed at beginning of time  step (m/s))
  braking strategy/1 -> [F_front_brake_req]
  config traction control/1(req'd force (N)) -> braking strategy/2, Sum/2, Relational Operator/1
  braking strategy/2 -> Sum/1, [F_rear_brake_req]
  Sum/1 -> [F_req_limited]
  Relational Operator/1 -> [slip_limited]
  [F_req] -> config traction control/3(total tractive force req'd (N))
  [F_req] -> Relational Operator/2
  [v_ave_req] -> config traction control/1(time-average vehicle speed  req'd (m/s))
  [v_ave_req] -> braking strategy/1
  front and rear brake controller (achievable)/2 -> [F_rear_brake]
  [F_max_rear_brake] -> front and rear brake controller (achievable)/5
  [F_max_front_brake] -> front and rear brake controller (achievable)/4
  [w_wheel_ach] -> front and rear brake controller (achievable)/3
  [F_drivetrain_ach] -> front and rear brake controller (achievable)/2
  front and rear brake controller (achievable)/1 -> [F_front_brake]
  [F_req] -> front and rear brake controller (achievable)/1
  gearbox control for series  HV and EV/1("gear number, out") -> [gear_number]
  gearbox control for series  HV and EV/2("gear ratio, out") -> [gear_ratio]
  gearbox control for series  HV and EV/3("shifting, out") -> [shifting]
  config traction control/4(weight on rear axle (N)) -> [wt_rear_axle]
  config traction control/5(front/total  traction ratio) -> [front_traction_ratio]
  Ground/1 -> front and rear brake controller (achievable)/6
